simulink model "cps_nozzle_control_v2"  (R2012b)
settings: Solver=FixedStepDiscrete  StartTime=0.0  StopTime=8.5  FixedStep=0.005  RelTol=1e-3
libraries: simulink x2
settings Model: RequirementInfo={} %GIDa_90988b37_44df_49de_baae_e1425c598f0e  Creator=pmosterm  LastModifiedBy=pmosterm
settings SolverCC: EnableConcurrentExecution=on  ConcurrentTasks=on
settings DataIOCC: SignalLoggingSaveFormat=ModelDataLogs  SaveOutput=off  SaveTime=off
settings OptimizationCC: InlineParams=on
settings DebuggingCC: UnderspecifiedInitializationDetection=Simplified  FcnCallInpInsideContextMsg=EnableAllAsWarning  ModelReferenceExtraNoncontSigs=warning
settings GRTTargetCC: CombineOutputUpdateFcns=off  GRTInterface=on
settings ConfigurationSet: Description=SimMechanics 2G

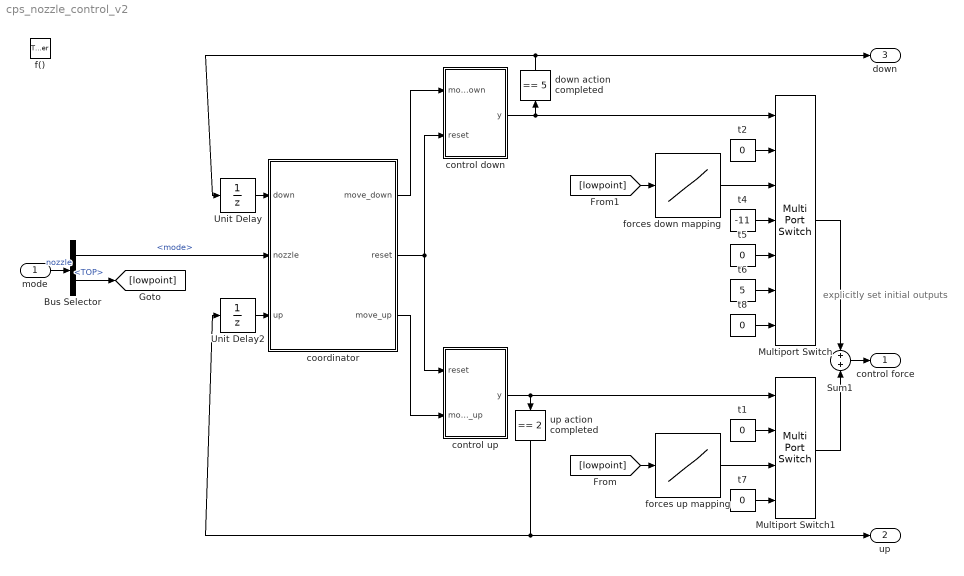
== system cps_nozzle_control_v2 ==
  note: explicitly
      | set initial
      | outputs
  mode : Inport  OutDataTypeStr=Bus:slBusNozzleOps  PortDimensions=1
  f() : TriggerPort  TriggerType=function-call  PortDimensions=1
  Bus Selector : BusSelector  OutputSignals=mode,TOP
  Multiport Switch : MultiPortSwitch  DataPortOrder=Zero-based contiguous  Inputs=6
  Multiport Switch1 : MultiPortSwitch  DataPortOrder=Zero-based contiguous
  Sum1 : Sum  Inputs=+|+
  Unit Delay : UnitDelay  SampleTime=-1
  Unit Delay2 : UnitDelay  SampleTime=-1
  control down : Stateflow chart  TreatAsAtomicUnit=on
  control up : Stateflow chart  TreatAsAtomicUnit=on
  coordinator : Stateflow chart  TreatAsAtomicUnit=on
  down action completed : simulink/Logic and Bit Operations/Compare To Constant  relop===  const=5  OutDataTypeStr=uint8
  forces down mapping : Lookup_n-D  NumberOfTableDimensions=1  BreakpointsForDimension1=[0:2]  Table=[-100 -80 -60]  RndMeth=Simplest  InputSameDT=on
  forces up mapping : Lookup_n-D  NumberOfTableDimensions=1  BreakpointsForDimension1=[0:2]  Table=[160 105 80]  RndMeth=Simplest  InputSameDT=on
  t{1..2,5,7..8} (5 alike) : Constant  Value=0  OutDataTypeStr=Inherit: Inherit via back propagation
  t4 : Constant  Value=-11  OutDataTypeStr=Inherit: Inherit via back propagation
  t6 : Constant  Value=5  OutDataTypeStr=Inherit: Inherit via back propagation
  up action completed : simulink/Logic and Bit Operations/Compare To Constant  relop===  const=2  OutDataTypeStr=uint8
  control force : Outport  OutDataTypeStr=double  PortDimensions=1  InitialOutput=0
  up : Outport  Port=2  OutDataTypeStr=uint8  PortDimensions=1  InitialOutput=0
  down : Outport  Port=3  OutDataTypeStr=uint8  PortDimensions=1  InitialOutput=0
  wires:
  t2/1 -> Multiport Switch/2
  forces down mapping/1 -> Multiport Switch/3
  t5/1 -> Multiport Switch/5
  t6/1 -> Multiport Switch/6
  control down/1(y) -> Multiport Switch/1, down action completed/1
  t8/1 -> Multiport Switch/7
  Multiport Switch/1 -> Sum1/1
  Sum1/1 -> control force/1
  control up/1(y) -> Multiport Switch1/1, up action completed/1
  down action completed/1 -> down/1, Unit Delay/1
  t1/1 -> Multiport Switch1/2
  t7/1 -> Multiport Switch1/4
  forces up mapping/1 -> Multiport Switch1/3
  Multiport Switch1/1 -> Sum1/2
  up action completed/1 -> Unit Delay2/1, up/1
  coordinator/1(move_down) -> control down/1(move_down)
  coordinator/3(move_up) -> control up/2(move_up)
  coordinator/2(reset) -> control down/2(reset), control up/1(reset)
  Unit Delay/1 -> coordinator/1(down)
  Unit Delay2/1 -> coordinator/3(up)
  mode/1 -> Bus Selector/1  "nozzle"
  Bus Selector/1 -> coordinator/2(nozzle)  "<mode>"
  Bus Selector/2 -> [lowpoint]  "<TOP>"
  t4/1 -> Multiport Switch/4
  [lowpoint] -> forces up mapping/1
  [lowpoint] -> forces down mapping/1

== stateflow chart cps_nozzle_control_v2/coordinator ==
  state neutral
  state move_down
  state reset
  state move_up
  state complete
  (default) -> neutral
  (junction 22) -> neutral : after(0.0025, sec)
  reset -> (junction 22)
  neutral -> move_down : [nozzle == NozzleOps.action]
  move_down -> move_up : [down]
  (junction 20) -> reset
  move_up -> complete : [up]
  complete -> (junction 20) : [nozzle != NozzleOps.action]
  data: down input; nozzle input; up input; move_down output boolean; reset output boolean; move_up output boolean

== stateflow chart cps_nozzle_control_v2/control down ==
  settings: executeAtInitialization=1
  state wait
    en:tref = 1e5;
    td = t - tref;
    y = 0;
  state operate
    en: tref = t;
    y = 1;
    du: td = t - tref;
    state S2
      en: y = 1;
    state S3
      en: y = 2;
    state S4
      en: y = 3;
    state S5
      en: y = 4;
    state S6
      en: y = 5;
    (default) -> S2
    S2 -> S3 : [td >= 0.25]/y=2;
    S3 -> S4 : [td >= 0.1]/y=3;
    S4 -> S5 : [td >= 0.3]/y=4;
    S5 -> S6 : [td >= 0.4]/y=5;
  (default) -> wait
  operate -> wait : [reset]
  wait -> operate : [move_down]
  data: y output; td local double; move_down input; reset input; tref local double

== stateflow chart cps_nozzle_control_v2/control up ==
  settings: executeAtInitialization=1
  state wait
    en: y = 0;
  state operate
    en: y = 1;
    state S2
      en: y = 1;
    state S3
      en: y = 2;
    (default) -> S2
    S2 -> S3 : after(0.19,sec)/y=2;
  (default) -> wait
  operate -> wait : [reset]
  wait -> operate : [move_up]
  data: reset input; y output; move_up input
